simulink model "discrete_sss_plant"  (R2019b)
settings: Solver=VariableStepAuto  StartTime=0.0  StopTime=20  RelTol=1e-3
settings Model: Creator=Murray  LastModifiedBy=Murray

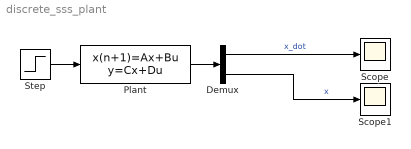
== system discrete_sss_plant ==
  Demux : Demux  Outputs=2
  Plant : DiscreteStateSpace  A="[0.9271  -0.4837;  0.09673  0.9755]"  B="[0.09673;  0.004897]"  C="[1  0;  0 1]"  D=[0; 0]  SampleTime=0.1
  Scope : Scope
  Scope1 : Scope
  Step : Step  SampleTime=0
  wires:
  Step/1 -> Plant/1
  Plant/1 -> Demux/1
  Demux/1 -> Scope/1  "x_dot"
  Demux/2 -> Scope1/1  "x"
